simulink model "lineFollowSim_real"  (R2022a)
settings: Solver=VariableStepAuto  StartTime=0.0  StopTime=10.0  RelTol=1e-3
undefined symbols (not defined in the file or in its folder): InputPWM, WheelSpeed
libraries: arduinolib x8, mobileRoboticsTrainingLib x1
settings Model: Creator=heath  LastModifiedBy=heath

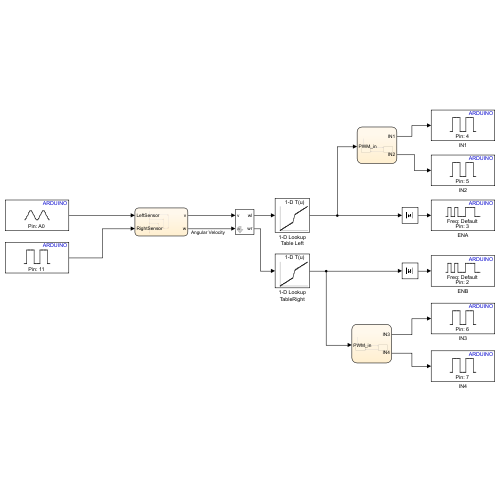
[thumbnail: Simulink's stored preview of the top-level diagram]
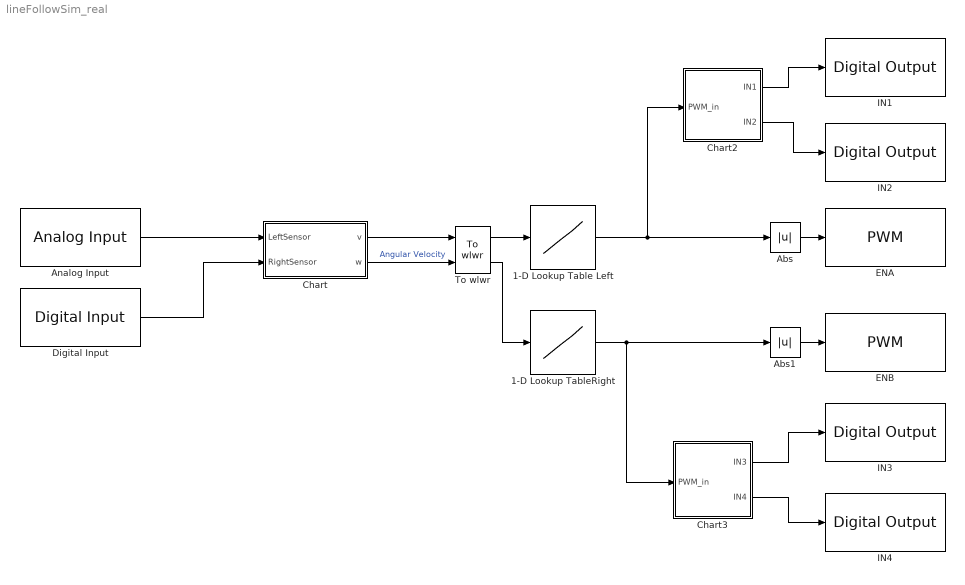
== system lineFollowSim_real ==
  1-D Lookup Table Left : Lookup_n-D  NumberOfTableDimensions=1  BreakpointsForDimension1=WheelSpeed  Table=InputPWM  InternalRulePriority=Speed  RndMeth=Simplest
  1-D Lookup TableRight : Lookup_n-D  NumberOfTableDimensions=1  BreakpointsForDimension1=WheelSpeed  Table=InputPWM  InternalRulePriority=Speed  RndMeth=Simplest
  Abs : Abs  SaturateOnIntegerOverflow=off
  Abs1 : Abs  SaturateOnIntegerOverflow=off
  Analog Input : arduinolib/Analog Input  pinNumber=0  ReadResultsOnly=off  ConversionTriggerSource=Software  ExternalTriggerType=uint32( 0 )  OutputDataType=uint16  EnableConversionCompleteNotify=off  EnableOuputStatus=off  SampleTime=-1  blockPlatform=arduino
  Chart : Stateflow chart  TreatAsAtomicUnit=on
  Chart2 : Stateflow chart  TreatAsAtomicUnit=on
  Chart3 : Stateflow chart  TreatAsAtomicUnit=on
  Digital Input : arduinolib/Digital Input  pinNumber=11  mode=Default  Direction=input  SampleTime=0.1  blockPlatform=arduino
  ENA : arduinolib/PWM  pinNumber=3  frequencyType=Default  desiredFrequency=490.2  achievableFrequency=490.2
  ENB : arduinolib/PWM  pinNumber=2  frequencyType=Default  desiredFrequency=490.2  achievableFrequency=490.2
  IN1 : arduinolib/Digital Output  pinNumber=4  Direction=output  blockPlatform=arduino
  IN2 : arduinolib/Digital Output  pinNumber=5  Direction=output  blockPlatform=arduino
  IN3 : arduinolib/Digital Output  pinNumber=6  Direction=output  blockPlatform=arduino
  IN4 : arduinolib/Digital Output  pinNumber=7  Direction=output  blockPlatform=arduino
  To wlwr : mobileRoboticsTrainingLib/To wlwr  axleLength=axleLength  wheelR=wheelR
  wires:
  Chart3/2(IN4) -> IN4/1
  Chart2/2(IN2) -> IN2/1
  Chart3/1(IN3) -> IN3/1
  To wlwr/1 -> 1-D Lookup Table Left/1
  Abs/1 -> ENA/1
  Chart2/1(IN1) -> IN1/1
  Abs1/1 -> ENB/1
  To wlwr/2 -> 1-D Lookup TableRight/1
  1-D Lookup Table Left/1 -> Chart2/1(PWM_in), Abs/1
  1-D Lookup TableRight/1 -> Chart3/1(PWM_in), Abs1/1
  Chart/1(v) -> To wlwr/1
  Chart/2(w) -> To wlwr/2  "Angular Velocity"
  Analog Input/1 -> Chart/1(LeftSensor)
  Digital Input/1 -> Chart/2(RightSensor)

== stateflow chart lineFollowSim_real/Chart3 ==
  state Forward
    entry:
    IN4 = 1;
    IN3 = 0;
  state Back
    entry:
    IN4 = 0;
    IN3 = 1;
  (default) -> Forward
  Forward -> Back : [PWM_in<0]
  Back -> Forward : [PWM_in>=0]
  data: PWM_in input; IN3 output; IN4 output

== stateflow chart lineFollowSim_real/Chart2 ==
  state Forward
    entry:
    IN1 = 1;
    IN2 = 0;
  state Back
    entry:
    IN1 = 0;
    IN2 = 1;
  (default) -> Forward
  Forward -> Back : [PWM_in<0]
  Back -> Forward : [PWM_in>=0]
  data: PWM_in input; IN1 output; IN2 output

== stateflow chart lineFollowSim_real/Chart ==
  (default) -> (junction 47) : % Movement
  (junction 47) -> (junction 48) [order 1] : [LeftSensor==3.3&&RightSensor==3.3]
  (junction 47) -> (junction 49) [order 2]
  (junction 48) -> (junction 56) : {v = 0; w = 0;}
  (junction 49) -> (junction 50) [order 1] : [LeftSensor==3.3]
  (junction 49) -> (junction 51) [order 2]
  (junction 50) -> (junction 55) : {v = 0.009; w = -0.1;}
  (junction 51) -> (junction 52) [order 1] : [RightSensor==3.3]
  (junction 51) -> (junction 53) [order 2] : {v = 0.009; w = 0;}
  (junction 52) -> (junction 54) : {v = 0.009; w = 0.1;}
  (junction 54) -> (junction 53)
  (junction 55) -> (junction 54)
  (junction 56) -> (junction 55)
  (junction 53) -> (junction 57)
  data: LeftSensor input; RightSensor input; v output; w output
